simulink model "VentilatorModel_v7"  (R2017b)
settings: Solver=ode23tb  StartTime=0.0  StopTime=30  FixedStep=0.001  MaxStep=0.005  RelTol=1e-7  EnableMultiTasking=on
values from neighbouring files (symbols this model uses):
  Mode = 1    [MainVentilator.m]
  SupplyPress_Air = 4000    [MainVentilator.m]
  SupplyPress_Oxigen = 2500    [MainVentilator.m]
  Throttle_Air = 0.8    [MainVentilator.m]
  Throttle_Oxigen = 1    [MainVentilator.m]
undefined symbols (not defined in the file or in its folder): BreathData, InputData
libraries: Simple_pneu_library x38, simulink x1
settings Model: SimulationMode=accelerator  Creator=ferossi  LastModifiedBy=ferossi
settings SolverCC: MaxConsecutiveMinStep=100  SolverResetMethod=Robust
settings DataIOCC: SaveFormat=Array
settings OptimizationCC: LifeSpan=inf
settings DebuggingCC: SolverPrmCheckMsg=warning  SFUnexpectedBacktrackingDiag=warning  SFNoUnconditionalDefaultTransitionDiag=warning  SFExecutionAtInitializationDiag=none
settings HardwareCC: ProdBitPerPointer=32  ProdBitPerSizeT=32  ProdBitPerPtrDiffT=32  ProdLargestAtomicFloat=None  ProdIntDivRoundTo=Undefined  ProdEndianess=Unspecified  ProdWordSize=32  ProdHWDeviceType=32-bit Generic
settings ModelReferenceCC: PropagateSignalLabelsOutOfModel=off
settings CodeAppCC: StateflowObjectComments=on
settings GRTTargetCC: TargetLangStandard=C89/C90 (ANSI)  GeneratePreprocessorConditionals=Disable all
settings ConfigComp: CovMetricSettings=dw  CovHtmlReporting=on  CovSaveCumulativeToWorkspaceVar=on  CovSaveSingleToWorkspaceVar=on  CovExternalEMLEnable=off  CovSFcnEnable=off

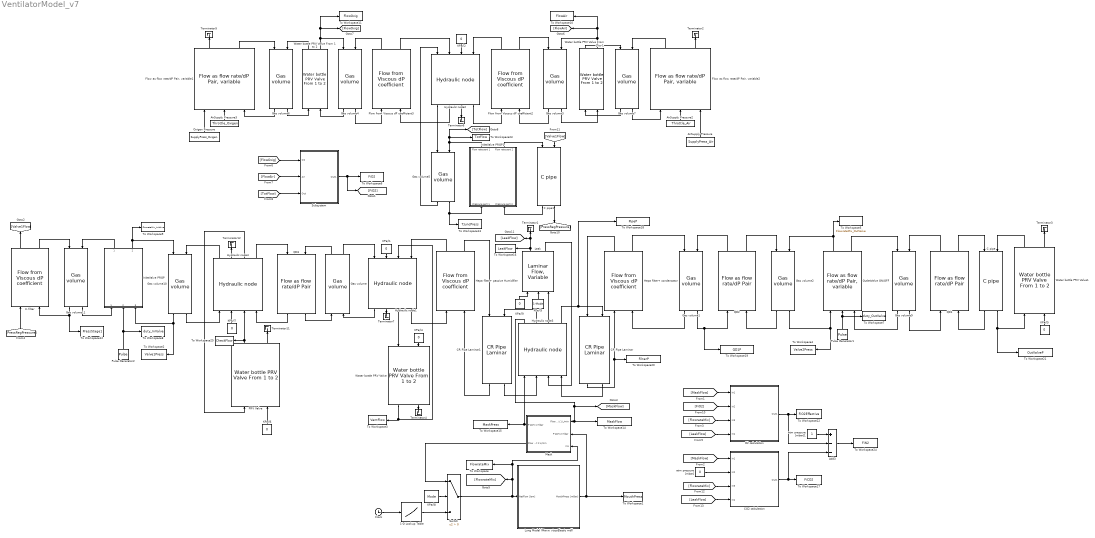
== system VentilatorModel_v7 ==
  1-D Lookup Table : Lookup_n-D  NumberOfTableDimensions=1  BreakpointsForDimension1=BreathData.Time  Table=BreathData.Flow  InternalRulePriority=Speed  RndMeth=Simplest  InputSameDT=on
  Add3 : Sum  Inputs=+--
  AirSupply Pressure : Constant  Value=SupplyPress_Air
  AirSupply Pressure2 : Constant  Value=Throttle_Air
  AirSupply Pressure3 : Constant  Value=Throttle_Oxigen
  C pipe : Simple_pneu_library/C pipe  p0=5  d=0.022  l=0.5
  C pipe1 : Simple_pneu_library/C pipe  p0=1000  d=0.022  l=0.5
  CO2 calculation : Subsystem
  CR Pipe Laminar : Simple_pneu_library/CR Pipe Laminar  d=0.022  L=1.5  mu=1.83E-5  P0=5
  CR Pipe Laminar1 : Simple_pneu_library/CR Pipe Laminar  d=0.022  L=1.5  mu=1.83E-5  P0=5
  Clock : Clock
  "Flow as flow rate/dP Pair, variable1" : Simple_pneu_library/Flow as flow rate//dP Pair, variable  dp=InputData.Regulator.BrkPress  flow=InputData.Regulator.Data
      mask Display: image('.\Pictures\ManReg.png');
  "Flow as flow rate/dP Pair, variable2" : Simple_pneu_library/Flow as flow rate//dP Pair, variable  dp=InputData.Regulator.BrkPress  flow=InputData.Regulator.Data
      mask Display: image('.\Pictures\ManReg.png');
  Flow from Viscous dP coefficient2 : Simple_pneu_library/Flow from Viscous dP  coefficient  Viscous_losses=1
  Flow from Viscous dP coefficient3 : Simple_pneu_library/Flow from Viscous dP  coefficient  Viscous_losses=1
  Gas volume{,1..2,9..10} (5 alike) : Simple_pneu_library/Gas volume  p0=5  Vol=0.1
  Gas volume11 : Simple_pneu_library/Gas volume  p0=1000  Vol=InputData.Stage2Volume
  Gas volume{3..4,6..7} (4 alike) : Simple_pneu_library/Gas volume  p0=0.8*min(SupplyPress_Air,SupplyPress_Oxigen)  Vol=0.1
  Gas volume5 : Simple_pneu_library/Gas volume  p0=0.8*min(SupplyPress_Air,SupplyPress_Oxigen)  Vol=InputData.Stage1Volume
  Hepa filter+ condensator : Simple_pneu_library/Flow from Viscous dP  coefficient  Viscous_losses=0.25+0.1
  Hepa filter+ passive Humidifier : Simple_pneu_library/Flow from Viscous dP  coefficient  Viscous_losses=0.25+0.01
  Hydraulic node{1..4} (4 alike) : Simple_pneu_library/Hydraulic node  SystemSampleTime=-1
      mask Display: image('.\Pictures\T-Junc.png');
  In filter : Simple_pneu_library/Flow from Viscous dP  coefficient  Viscous_losses=0.025
  InletValve PROP : Subsystem  mask{dp=InputData.InValve.BrkPress, flow=InputData.InValve.Data, posizione=InputData.InValve.BrkDuty}
      mask prompts: dp "Reference Pressure Drop [mbar]"; flow "Flow Rate [L/min]"; posizione "Duty [%]"
      mask Display: image('.\Pictures\CamozziPROP.png');
  InletValve PROP1 : Subsystem  mask{dp=InputData.PReg.BrkPress, flow=InputData.PReg.Data}
      mask prompts: dp "Reference Pressure Drop [mbar]"; flow "Flow Rate [L/min]"
      mask Display: image('.\Pictures\CamozziPReg.png');
  KPa/l{1..2,4..7,9} (7 alike) : Constant  Value=0
  KPa/l3 : Constant  Value=1-Mode
  KPa/l8 : Constant  Value=Mode
  Leak : Simple_pneu_library/Laminar Flow, Variable  Viscous_losses=60
  Lung Model (Maxw viscoElastic mdl) : Subsystem  mask{Stiff1=100, Stiff2=2.6, Damp=0.9, R0=0.47, Kv=-0.45, Kf=0.01}
      mask prompts: Stiff1 "Stiffness in series with damp"; Stiff2 "Stiffness in parallel"; Damp "Damping"; R0 "Laminar flow resistance"; Kv "Volum resistance coeff"; Kf "Flow resistance coeff"
      mask Display: image('.\Pictures\Lung.PNG');
  Mask : Subsystem  mask{vol=InputData.MaskVolume, P0=5, d=0.022, rho=1.225}
      mask prompts: vol "Volume [L]"; P0 "Initial condition [mbar]"; d "Diameter [m]"; rho "Density [kg/m3]"
      mask Display: image('.\Pictures\Mascherina.jpg');
  O2 calculation : Subsystem
  OutletValve ON/OFF : Simple_pneu_library/Flow as flow rate//dP Pair, variable  dp=InputData.OutValve.BrkPress  flow=InputData.OutValve.Data
      mask Display: image('.\Pictures\CamozziONOFF.png');
  Oxigen Pressure : Constant  Value=SupplyPress_Oxigen
  PRV Valve : Simple_pneu_library/Water bottle PRV Valve From 1 to 2  Viscous_losses=0.1  Crack=80  Delay=0.001
      mask Display: image('.\Pictures\PeepValve.png');
  Pulse Generator1 : DiscretePulseGenerator  PulseType=Time based  Amplitude=InputData.OutValve.DutyMax  Period=InputData.InValve.Period  PulseWidth=InputData.OutValve.PulseWidth  PhaseDelay=2.1
  Pulse Generator2 : DiscretePulseGenerator  PulseType=Time based  Amplitude=InputData.InValve.DutyMax  Period=InputData.InValve.Period  PulseWidth=InputData.InValve.PulseWidth
  QD1 : Simple_pneu_library/Flow as  flow rate//dP Pair  dp=20  flow=160
      mask Display: image('.\Pictures\QD.png');
  QD2 : Simple_pneu_library/Flow as  flow rate//dP Pair  dp=20  flow=160
      mask Display: image('.\Pictures\QD.png');
  QD3 : Simple_pneu_library/Flow as  flow rate//dP Pair  dp=20  flow=160
      mask Display: image('.\Pictures\QD.png');
  Subsystem : Subsystem
  Switch : Switch  Criteria=u2 > Threshold
  Terminator{1..7,11..12} (9 alike) : Terminator
  To Workspace : ToWorkspace  VariableName=FlowrateMix  SampleTime=-1
  To Workspace1 : ToWorkspace  VariableName=MouthPress  SampleTime=-1
  To Workspace10 : ToWorkspace  VariableName=FlowAir  SampleTime=-1
  To Workspace11 : ToWorkspace  VariableName=FlowOxig  SampleTime=-1
  To Workspace12 : ToWorkspace  VariableName=PressStage1  SampleTime=-1
  To Workspace13 : ToWorkspace  VariableName=TJuncPress  SampleTime=-1
  To Workspace14 : ToWorkspace  VariableName=MaskFlow  SampleTime=-1
  To Workspace15 : ToWorkspace  VariableName=MaskPress  SampleTime=-1
  To Workspace16 : ToWorkspace  VariableName=LeakFlow  SampleTime=-1
  To Workspace17 : ToWorkspace  VariableName=FiCO2  SampleTime=-1
  To Workspace18 : ToWorkspace  VariableName=PipeP  SampleTime=-1
  To Workspace19 : ToWorkspace  VariableName=QD1P  SampleTime=-1
  To Workspace2 : ToWorkspace  VariableName=Valve1Press  SampleTime=-1
  To Workspace20 : ToWorkspace  VariableName=FilterP  SampleTime=-1
  To Workspace21 : ToWorkspace  VariableName=OutValveP  SampleTime=-1
  To Workspace22 : ToWorkspace  VariableName=FiO2Effective  SampleTime=-1
  To Workspace23 : ToWorkspace  VariableName=TotFlow  SampleTime=-1
  To Workspace24 : ToWorkspace  VariableName=FiN2  SampleTime=-1
  To Workspace25 : ToWorkspace  VariableName=CheckFlow  SampleTime=-1
  To Workspace3 : ToWorkspace  VariableName=VentFlow  SampleTime=-1
  To Workspace4 : ToWorkspace  VariableName=Valve2Press  SampleTime=-1
  To Workspace5 : ToWorkspace  VariableName=FlowrateMix_OutValve  SampleTime=-1
  To Workspace6 : ToWorkspace  VariableName=FiO2  SampleTime=-1
  To Workspace7 : ToWorkspace  VariableName=duty_OutValve  SampleTime=-1
  To Workspace8 : ToWorkspace  VariableName=duty_InValve  SampleTime=-1
  To Workspace9 : ToWorkspace  VariableName=FlowrateMix_InValve  SampleTime=-1
  "Water bottle PRV Valve " : Simple_pneu_library/Water bottle PRV Valve From 1 to 2  Viscous_losses=0.1  Crack=30  Delay=0.001
      mask Display: image('.\Pictures\VentValveBottle.png');
  Water bottle PRV Valve From 1 to 1 : Simple_pneu_library/Water bottle PRV Valve From 1 to 2  Viscous_losses=0.1  Crack=1  Delay=0.001
      mask Display: image('.\Pictures\NRV.png');
  Water bottle PRV Valve From 1 to 2 : Simple_pneu_library/Water bottle PRV Valve From 1 to 2  Viscous_losses=0.1  Crack=1  Delay=0.001
      mask Display: image('.\Pictures\NRV.png');
  Water bottle PRV Valve1 : Simple_pneu_library/Water bottle PRV Valve From 1 to 2  Viscous_losses=0.1  Crack=5  Delay=0.001
      mask Display: image('.\Pictures\PeepValve.png');
  atm pressure [mbar] : Constant  Value=0
  atm pressure [mbar]1 : Constant
  wires:
  Lung Model (Maxw viscoElastic mdl)/1(MouthPress [mBar]) -> Mask/2(P port 2 mbar), To Workspace1/1
  Pulse Generator1/1 -> To Workspace7/1, OutletValve ON/OFF/2
  [PressRegPressure] -> In filter/1
  "Water bottle PRV Valve "/2 -> Terminator4/1
  "Water bottle PRV Valve "/1 -> Hydraulic node1/3, To Workspace3/1
  Hydraulic node1/3 -> "Water bottle PRV Valve "/1
  KPa/l4/1 -> "Water bottle PRV Valve "/2
  Water bottle PRV Valve1/2 -> Terminator3/1
  Water bottle PRV Valve1/1 -> C pipe/2
  KPa/l5/1 -> Water bottle PRV Valve1/2
  C pipe/2 -> Water bottle PRV Valve1/1, To Workspace21/1
  AirSupply Pressure2/1 -> "Flow as flow rate/dP Pair, variable2"/2
  "Flow as flow rate/dP Pair, variable2"/2 -> Terminator2/1
  AirSupply Pressure3/1 -> "Flow as flow rate/dP Pair, variable1"/2
  Oxigen Pressure/1 -> "Flow as flow rate/dP Pair, variable1"/1
  "Flow as flow rate/dP Pair, variable1"/1 -> Terminator5/1
  Flow from Viscous dP coefficient2/2 -> Gas volume3/1
  Gas volume3/1 -> Flow from Viscous dP coefficient2/2
  Flow from Viscous dP coefficient3/1 -> Gas volume4/2
  Gas volume4/2 -> Flow from Viscous dP coefficient3/1
  Hydraulic node2/2 -> Flow from Viscous dP coefficient3/2
  Flow from Viscous dP coefficient3/2 -> Hydraulic node2/2
  Hydraulic node2/4 -> Flow from Viscous dP coefficient2/1
  Hydraulic node2/3 -> Terminator6/1
  KPa/l2/1 -> Hydraulic node2/3
  Hydraulic node2/1 -> Gas volume5/1
  Flow from Viscous dP coefficient2/1 -> Hydraulic node2/4
  Pulse Generator2/1 -> InletValve PROP/2(Valve position), To Workspace8/1
  [Valve1Flow] -> C pipe1/2
  AirSupply Pressure/1 -> "Flow as flow rate/dP Pair, variable2"/3
  InletValve PROP1/2("Flow rate port 2 ") -> C pipe1/1
  C pipe1/2 -> [PressRegPressure]
  CR Pipe Laminar1/2 -> Hydraulic node3/2
  CR Pipe Laminar1/1 -> Hepa filter+ passive Humidifier/2
  Hepa filter+ passive Humidifier/2 -> CR Pipe Laminar1/1
  Hydraulic node3/2 -> CR Pipe Laminar1/2
  Hydraulic node3/4 -> To Workspace18/1, CR Pipe Laminar/2
  Hepa filter+ condensator/1 -> CR Pipe Laminar/1
  CR Pipe Laminar/1 -> Hepa filter+ condensator/1, To Workspace20/1
  CR Pipe Laminar/2 -> Hydraulic node3/4
  QD1/2 -> C pipe/1
  QD1/1 -> Gas volume9/2
  OutletValve ON/OFF/2 -> Gas volume9/1
  Gas volume9/1 -> OutletValve ON/OFF/3
  C pipe/1 -> QD1/2
  QD2/2 -> Gas volume2/1
  Gas volume2/1 -> QD2/2
  Gas volume2/2 -> To Workspace4/1, OutletValve ON/OFF/1
  QD2/1 -> Gas volume1/2
  Gas volume1/2 -> To Workspace19/1, QD2/1
  OutletValve ON/OFF/1 -> To Workspace5/1, Gas volume2/2
  Hepa filter+ condensator/2 -> Gas volume1/1
  Gas volume1/1 -> Hepa filter+ condensator/2
  Hydraulic node1/4 -> Hepa filter+ passive Humidifier/1
  Hepa filter+ passive Humidifier/1 -> Hydraulic node1/4
  KPa/l1/1 -> Hydraulic node1/2
  Hydraulic node1/2 -> Terminator7/1
  Gas volume/1 -> QD3/2
  Gas volume/2 -> Hydraulic node1/1
  QD3/2 -> Gas volume/1
  Hydraulic node4/4 -> QD3/1
  KPa/l6/1 -> PRV Valve/2
  PRV Valve/1 -> To Workspace25/1, Hydraulic node4/3
  KPa/l7/1 -> Hydraulic node4/2
  Hydraulic node4/2 -> Terminator12/1
  Hydraulic node1/1 -> Gas volume/2
  Hydraulic node4/3 -> PRV Valve/1
  Gas volume10/2 -> Hydraulic node4/1
  PRV Valve/2 -> Terminator11/1
  Hydraulic node4/1 -> Gas volume10/2
  QD3/1 -> Hydraulic node4/4
  Gas volume10/1 -> To Workspace2/1, InletValve PROP/3(Pressure port 2)
  InletValve PROP1/1("Flow rate port 1 ") -> To Workspace23/1, [TotFlow], Gas volume5/2
  Gas volume5/1 -> Hydraulic node2/1
  Gas volume5/2 -> To Workspace13/1, InletValve PROP1/1("Pressure port 1 ")
  C pipe1/1 -> InletValve PROP1/2(Pressure port 2)
  In filter/1 -> [Valve1Flow]
  Gas volume11/2 -> InletValve PROP/1("Pressure port 1 ")
  Gas volume11/1 -> To Workspace12/1, In filter/2
  InletValve PROP/1("Flow rate port 1 ") -> Gas volume11/2
  In filter/2 -> Gas volume11/1
  InletValve PROP/2("Flow rate port 2 ") -> Gas volume10/1, To Workspace9/1
  Water bottle PRV Valve From 1 to 2/2 -> [FlowOxig], To Workspace11/1, Gas volume4/1
  Gas volume4/1 -> Water bottle PRV Valve From 1 to 2/2
  Water bottle PRV Valve From 1 to 2/1 -> Gas volume6/2
  Gas volume6/2 -> Water bottle PRV Valve From 1 to 2/1
  Gas volume6/1 -> "Flow as flow rate/dP Pair, variable1"/3
  "Flow as flow rate/dP Pair, variable1"/2 -> Gas volume6/1
  Gas volume7/2 -> "Flow as flow rate/dP Pair, variable2"/1
  "Flow as flow rate/dP Pair, variable2"/1 -> Gas volume7/2
  Gas volume9/2 -> QD1/1
  KPa/l8/1 -> Switch/2
  1-D Lookup Table/1 -> Switch/3
  Clock/1 -> 1-D Lookup Table/1
  Switch/1 -> Mask/3(In1), To Workspace/1, [FlowrateMix], Lung Model (Maxw viscoElastic mdl)/1(NetFlow [lpm])
  Mask/2(Flow port 2 L/min) -> Switch/1
  Mask/1(P port 1 mbar) -> To Workspace15/1, Hydraulic node3/1
  Hydraulic node3/1 -> To Workspace14/1, Mask/1(Flow port 1 L/min), [MaskFlow]
  KPa/l3/1 -> Leak/2
  Hydraulic node3/3 -> Leak/3
  Leak/2 -> Hydraulic node3/3
  Leak/1 -> To Workspace16/1, [LeakFlow], Terminator1/1
  KPa/l9/1 -> Leak/1
  Subsystem/1(Out1) -> To Workspace6/1, [FiO2]
  [FlowOxig] -> Subsystem/1(O2)
  [FlowAir] -> Subsystem/2(Air)
  [TotFlow] -> Subsystem/3(Out)
  Water bottle PRV Valve From 1 to 1/2 -> [FlowAir], To Workspace10/1, Gas volume3/2
  Water bottle PRV Valve From 1 to 1/1 -> Gas volume7/1
  Gas volume7/1 -> Water bottle PRV Valve From 1 to 1/1
  Gas volume3/2 -> Water bottle PRV Valve From 1 to 1/2
  [MaskFlow] -> O2 calculation/1(In1)
  [FiO2] -> O2 calculation/2(In2)
  [FlowrateMix] -> O2 calculation/3(In3)
  [LeakFlow] -> O2 calculation/4(In4)
  O2 calculation/1(Out1) -> Add3/2, To Workspace22/1
  atm pressure [mbar]/1 -> CO2 calculation/2(In2)
  CO2 calculation/1(Out1) -> Add3/3, To Workspace17/1
  [MaskFlow] -> CO2 calculation/1(In1)
  [FlowrateMix] -> CO2 calculation/3(In3)
  [LeakFlow] -> CO2 calculation/4(In4)
  atm pressure [mbar]1/1 -> Add3/1
  Add3/1 -> To Workspace24/1

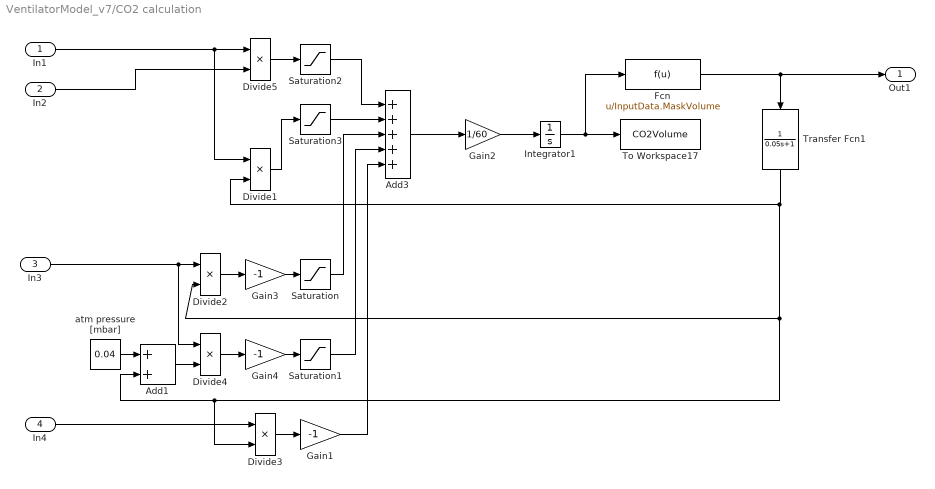
== system VentilatorModel_v7/CO2 calculation ==
  In1 : Inport
  In2 : Inport  Port=2
  In3 : Inport  Port=3
  In4 : Inport  Port=4
  Add1 : Sum
  Add3 : Sum  Inputs=+++++
  Divide{1..5} (5 alike) : Product  Inputs=**
  Fcn : Fcn  Expr=u/InputData.MaskVolume
  Gain1 : Gain  Gain=-1
  Gain2 : Gain  Gain=1/60
  Gain3 : Gain  Gain=-1
  Gain4 : Gain  Gain=-1
  Integrator1 : Integrator
  Saturation : Saturate  UpperLimit=0  LowerLimit=-200
  Saturation1 : Saturate  UpperLimit=150  LowerLimit=0
  Saturation2 : Saturate  UpperLimit=200  LowerLimit=0
  Saturation3 : Saturate  UpperLimit=0  LowerLimit=-200
  To Workspace17 : ToWorkspace  VariableName=CO2Volume  SampleTime=-1
  Transfer Fcn1 : TransferFcn  Denominator=[0.05 1]
  atm pressure [mbar] : Constant  Value=0.04
  Out1 : Outport
  wires:
  Saturation1/1 -> Add3/4
  Saturation/1 -> Add3/3
  Gain3/1 -> Saturation/1
  In3/1 -> Divide4/1, Divide2/1
  Gain4/1 -> Saturation1/1
  Divide4/1 -> Gain4/1
  Gain1/1 -> Add3/5
  Gain2/1 -> Integrator1/1
  Add3/1 -> Gain2/1
  In2/1 -> Divide5/2
  atm pressure [mbar]/1 -> Add1/1
  Divide2/1 -> Gain3/1
  Fcn/1 -> Out1/1, Transfer Fcn1/1
  In4/1 -> Divide3/1
  Divide3/1 -> Gain1/1
  In1/1 -> Divide1/1, Divide5/1
  Divide1/1 -> Saturation3/1
  Saturation3/1 -> Add3/2
  Add1/1 -> Divide4/2
  Integrator1/1 -> Fcn/1, To Workspace17/1
  Transfer Fcn1/1 -> Divide1/2, Divide2/2, Add1/2, Divide3/2
  Saturation2/1 -> Add3/1
  Divide5/1 -> Saturation2/1

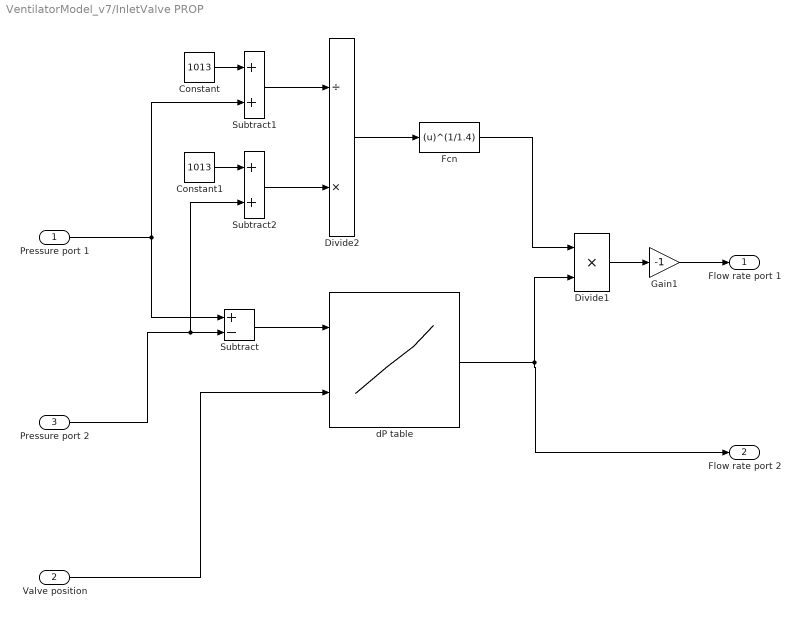
== system VentilatorModel_v7/InletValve PROP ==
  "Pressure port 1 " : Inport
  Valve position : Inport  Port=2
  Pressure port 2 : Inport  Port=3
  Constant : Constant  Value=1013
  Constant1 : Constant  Value=1013
  Divide1 : Product  Inputs=**
  Divide2 : Product  Inputs=/*
  Fcn : Fcn  Expr=(u)^(1/1.4)
  Gain1 : Gain  Gain=-1
  Subtract : Sum  Inputs=+-
  Subtract1 : Sum
  Subtract2 : Sum
  dP table : Lookup_n-D  BreakpointsForDimension1=dp  BreakpointsForDimension2=posizione  BeginIndexSearchUsingPreviousIndexResult=on  Table=flow  InternalRulePriority=Speed  RndMeth=Simplest  InputSameDT=on
  "Flow rate port 1 " : Outport
  "Flow rate port 2 " : Outport  Port=2
  wires:
  Valve position/1 -> dP table/2
  Pressure port 2/1 -> Subtract2/2, Subtract/2
  Gain1/1 -> "Flow rate port 1 "/1
  Subtract/1 -> dP table/1
  "Pressure port 1 "/1 -> Subtract/1, Subtract1/2
  dP table/1 -> "Flow rate port 2 "/1, Divide1/2
  Constant/1 -> Subtract1/1
  Constant1/1 -> Subtract2/1
  Subtract1/1 -> Divide2/1
  Subtract2/1 -> Divide2/2
  Divide2/1 -> Fcn/1
  Divide1/1 -> Gain1/1
  Fcn/1 -> Divide1/1

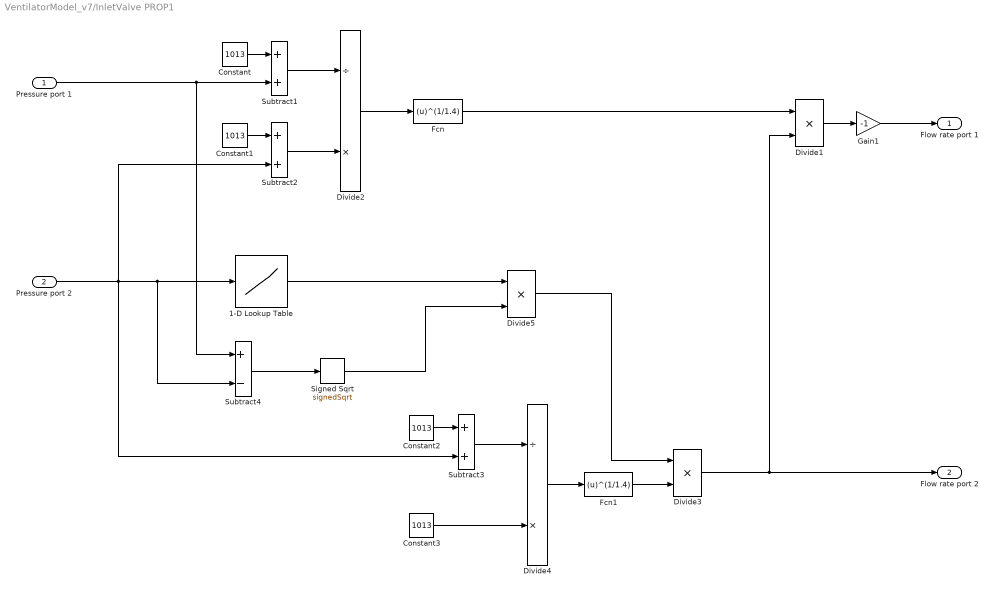
== system VentilatorModel_v7/InletValve PROP1 ==
  "Pressure port 1 " : Inport
  Pressure port 2 : Inport  Port=2
  1-D Lookup Table : Lookup_n-D  NumberOfTableDimensions=1  BreakpointsForDimension1=dp  Table=flow  ExtrapMethod=Clip  InternalRulePriority=Speed  RndMeth=Simplest  InputSameDT=on
  Constant{,1..3} (4 alike) : Constant  Value=1013
  Divide1 : Product  Inputs=**
  Divide2 : Product  Inputs=/*
  Divide3 : Product  Inputs=**
  Divide4 : Product  Inputs=/*
  Divide5 : Product  Inputs=**
  Fcn : Fcn  Expr=(u)^(1/1.4)
  Fcn1 : Fcn  Expr=(u)^(1/1.4)
  Gain1 : Gain  Gain=-1
  Signed Sqrt : Sqrt  Operator=signedSqrt  SaturateOnIntegerOverflow=on
  Subtract1 : Sum
  Subtract2 : Sum
  Subtract3 : Sum
  Subtract4 : Sum  Inputs=+-
  "Flow rate port 1 " : Outport
  "Flow rate port 2 " : Outport  Port=2
  wires:
  Gain1/1 -> "Flow rate port 1 "/1
  Subtract2/1 -> Divide2/2
  Divide2/1 -> Fcn/1
  "Pressure port 1 "/1 -> Subtract4/1, Subtract1/2
  Constant/1 -> Subtract1/1
  Subtract1/1 -> Divide2/1
  Pressure port 2/1 -> Subtract4/2, 1-D Lookup Table/1, Subtract2/2, Subtract3/2
  Constant1/1 -> Subtract2/1
  Fcn/1 -> Divide1/1
  Divide1/1 -> Gain1/1
  Constant2/1 -> Subtract3/1
  Subtract3/1 -> Divide4/1
  Divide4/1 -> Fcn1/1
  Fcn1/1 -> Divide3/2
  Constant3/1 -> Divide4/2
  Divide3/1 -> "Flow rate port 2 "/1, Divide1/2
  1-D Lookup Table/1 -> Divide5/1
  Subtract4/1 -> Signed Sqrt/1
  Signed Sqrt/1 -> Divide5/2
  Divide5/1 -> Divide3/1

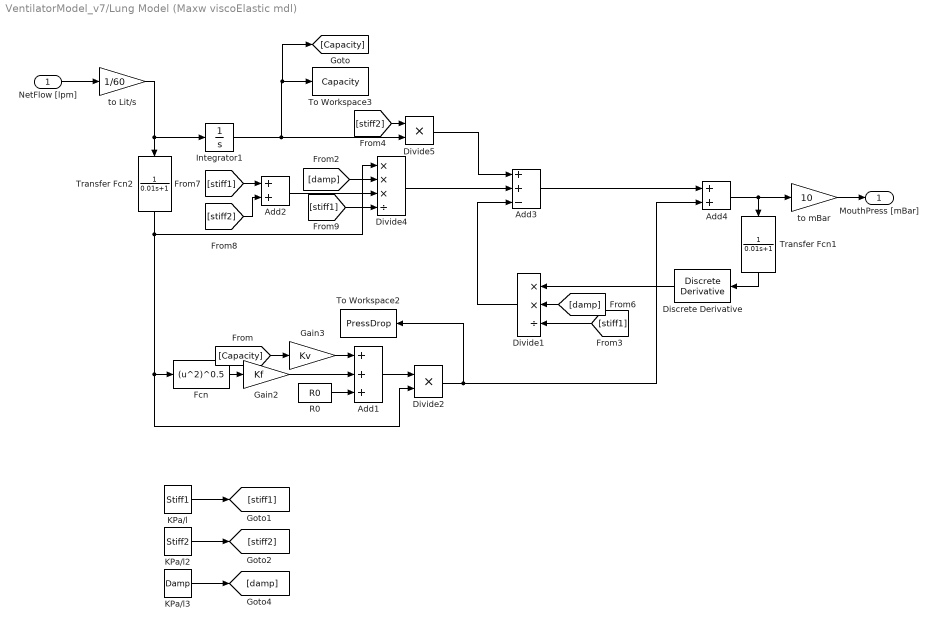
== system VentilatorModel_v7/Lung Model (Maxw viscoElastic mdl) ==
  NetFlow [lpm] : Inport
  Add1 : Sum  Inputs=+++
  Add2 : Sum
  Add3 : Sum  Inputs=++-
  Add4 : Sum
  Discrete Derivative : simulink/Discrete/Discrete Derivative  gainval=1.0  ICPrevScaledInput=0.0  OutMin=[]  OutMax=[]  OutDataType=fixdt(1, 16)  OutScaling=2^-10  DoSatur=off
  Divide1 : Product  Inputs=**/
  Divide2 : Product  Inputs=**
  Divide4 : Product  Inputs=***/
  Divide5 : Product  Inputs=**
  Fcn : Fcn  Expr=(u^2)^0.5
  Gain2 : Gain  Gain=Kf
  Gain3 : Gain  Gain=Kv
  Integrator1 : Integrator
  KPa/l : Constant  Value=Stiff1
  KPa/l2 : Constant  Value=Stiff2
  KPa/l3 : Constant  Value=Damp
  R0 : Constant  Value=R0
  To Workspace2 : ToWorkspace  VariableName=PressDrop  SampleTime=-1
  To Workspace3 : ToWorkspace  VariableName=Capacity  SampleTime=-1
  Transfer Fcn1 : TransferFcn  Denominator=[0.01 1]
  Transfer Fcn2 : TransferFcn  Denominator=[0.01 1]
  to Lit/s : Gain  Gain=1/60
  to mBar : Gain  Gain=10
  MouthPress [mBar] : Outport
  wires:
  NetFlow [lpm]/1 -> to Lit/s/1
  Add3/1 -> Add4/1
  Add4/1 -> Transfer Fcn1/1, to mBar/1
  KPa/l3/1 -> [damp]
  R0/1 -> Add1/3
  KPa/l/1 -> [stiff1]
  Fcn/1 -> Gain2/1
  Gain3/1 -> Add1/1
  Add1/1 -> Divide2/1
  [stiff1] -> Add2/1
  Gain2/1 -> Add1/2
  [damp] -> Divide1/2
  Divide5/1 -> Add3/1
  [stiff1] -> Divide1/3
  [stiff2] -> Add2/2
  Divide2/1 -> Add4/2, To Workspace2/1
  [stiff1] -> Divide4/4
  Divide1/1 -> Add3/3
  Divide4/1 -> Add3/2
  Integrator1/1 -> Divide5/2, [Capacity], To Workspace3/1
  [damp] -> Divide4/2
  Discrete Derivative/1 -> Divide1/1
  [stiff2] -> Divide5/1
  KPa/l2/1 -> [stiff2]
  [Capacity] -> Gain3/1
  Add2/1 -> Divide4/3
  to mBar/1 -> MouthPress [mBar]/1
  Transfer Fcn1/1 -> Discrete Derivative/1
  to Lit/s/1 -> Transfer Fcn2/1, Integrator1/1
  Transfer Fcn2/1 -> Fcn/1, Divide2/2, Divide4/1

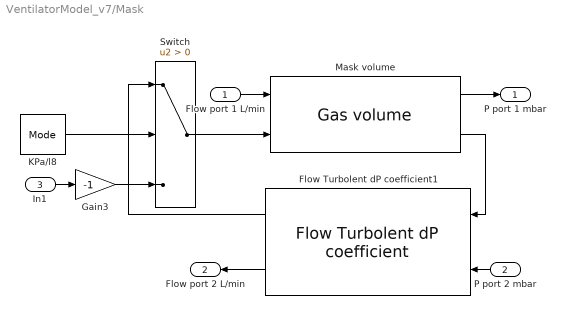
== system VentilatorModel_v7/Mask ==
  Flow port 1 L/min : Inport
  P port 2 mbar : Inport  Port=2
  In1 : Inport  Port=3
  Flow Turbolent dP coefficient1 : Simple_pneu_library/Flow Turbolent dP coefficient  cq=100  d=d  rho=rho
  Gain3 : Gain  Gain=-1
  KPa/l8 : Constant  Value=Mode
  Mask volume : Simple_pneu_library/Gas volume  p0=P0  Vol=vol
  Switch : Switch  Criteria=u2 > Threshold
  P port 1 mbar : Outport
  Flow port 2 L/min : Outport  Port=2
  wires:
  Flow Turbolent dP coefficient1/2 -> Flow port 2 L/min/1
  Mask volume/2 -> Flow Turbolent dP coefficient1/1
  P port 2 mbar/1 -> Flow Turbolent dP coefficient1/2
  Flow port 1 L/min/1 -> Mask volume/1
  Mask volume/1 -> P port 1 mbar/1
  KPa/l8/1 -> Switch/2
  Switch/1 -> Mask volume/2
  Flow Turbolent dP coefficient1/1 -> Switch/1
  In1/1 -> Gain3/1
  Gain3/1 -> Switch/3

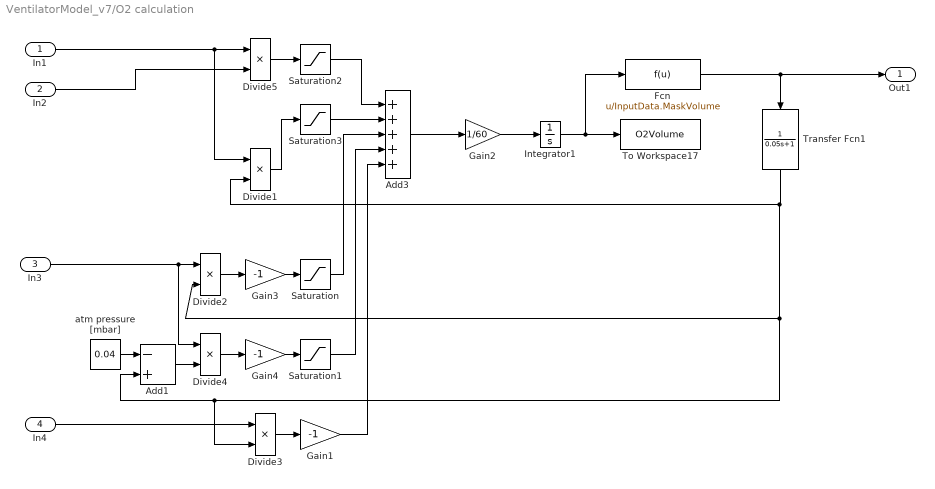
== system VentilatorModel_v7/O2 calculation ==
  In1 : Inport
  In2 : Inport  Port=2
  In3 : Inport  Port=3
  In4 : Inport  Port=4
  Add1 : Sum  Inputs=-+
  Add3 : Sum  Inputs=+++++
  Divide{1..5} (5 alike) : Product  Inputs=**
  Fcn : Fcn  Expr=u/InputData.MaskVolume
  Gain1 : Gain  Gain=-1
  Gain2 : Gain  Gain=1/60
  Gain3 : Gain  Gain=-1
  Gain4 : Gain  Gain=-1
  Integrator1 : Integrator  InitialCondition=InputData.MaskVolume*InputData.FiO2Target
  Saturation : Saturate  UpperLimit=0  LowerLimit=-200
  Saturation1 : Saturate  UpperLimit=150  LowerLimit=0
  Saturation2 : Saturate  UpperLimit=200  LowerLimit=0
  Saturation3 : Saturate  UpperLimit=0  LowerLimit=-200
  To Workspace17 : ToWorkspace  VariableName=O2Volume  SampleTime=-1
  Transfer Fcn1 : TransferFcn  Denominator=[0.05 1]
  atm pressure [mbar] : Constant  Value=0.04
  Out1 : Outport
  wires:
  Saturation1/1 -> Add3/4
  Saturation/1 -> Add3/3
  Gain3/1 -> Saturation/1
  In3/1 -> Divide4/1, Divide2/1
  Gain4/1 -> Saturation1/1
  Divide4/1 -> Gain4/1
  Gain1/1 -> Add3/5
  Gain2/1 -> Integrator1/1
  Add3/1 -> Gain2/1
  In2/1 -> Divide5/2
  atm pressure [mbar]/1 -> Add1/1
  Divide2/1 -> Gain3/1
  Fcn/1 -> Out1/1, Transfer Fcn1/1
  In4/1 -> Divide3/1
  Divide3/1 -> Gain1/1
  In1/1 -> Divide1/1, Divide5/1
  Divide1/1 -> Saturation3/1
  Saturation3/1 -> Add3/2
  Add1/1 -> Divide4/2
  Integrator1/1 -> Fcn/1, To Workspace17/1
  Transfer Fcn1/1 -> Divide1/2, Divide2/2, Add1/2, Divide3/2
  Saturation2/1 -> Add3/1
  Divide5/1 -> Saturation2/1

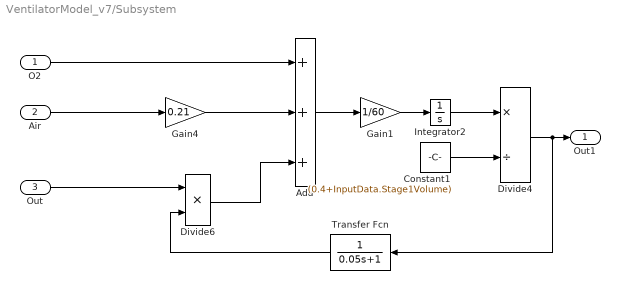
== system VentilatorModel_v7/Subsystem ==
  O2 : Inport
  Air : Inport  Port=2
  Out : Inport  Port=3
  Add : Sum  Inputs=+++
  Constant1 : Constant  Value=(0.4+InputData.Stage1Volume)
  Divide4 : Product  Inputs=*/
  Divide6 : Product  Inputs=**
  Gain1 : Gain  Gain=1/60
  Gain4 : Gain  Gain=0.21
  Integrator2 : Integrator  InitialCondition=(0.4+InputData.Stage1Volume)*InputData.FiO2Target
  Transfer Fcn : TransferFcn  Denominator=[0.05 1]
  Out1 : Outport
  wires:
  Transfer Fcn/1 -> Divide6/2
  Gain1/1 -> Integrator2/1
  Add/1 -> Gain1/1
  Gain4/1 -> Add/2
  O2/1 -> Add/1
  Air/1 -> Gain4/1
  Divide4/1 -> Transfer Fcn/1, Out1/1
  Divide6/1 -> Add/3
  Constant1/1 -> Divide4/2
  Integrator2/1 -> Divide4/1
  Out/1 -> Divide6/1
